simulink model "Wind_App"  (R2020a)
settings: Solver=VariableStepAuto  StartTime=0.0  StopTime=10  RelTol=1e-3
undefined symbols (not defined in the file): D1, D11, Delta
libraries: powerlib x15, re_lib x1
settings Model: Creator=royde  LastModifiedBy=royde

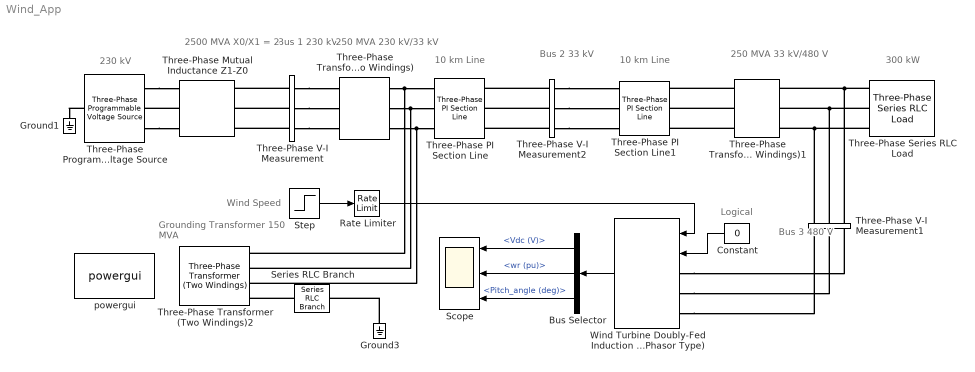
== system Wind_App ==
  note: Bus 1
      | 230 kV
  note: 230 kV
  note: 2500 MVA
      | X0/X1 = 2
  note: 250 MVA
      | 230 kV/33 kV
  note: 250 MVA
      | 33 kV/480 V
  note: Bus 3
      | 480 V
  note: 300 kW
  note: Wind Speed
  note: Logical
  note: Bus 2
      | 33 kV
  note: 10 km Line
  note: 10 km Line
  note: Grounding Transformer
      | 150 MVA
  Bus Selector : BusSelector  OutputSignals=Vdc (V),wr (pu),Pitch_angle (deg)
  Constant : Constant  Value=0
  Ground1 : powerlib/Elements/Ground  LConnTagsString=a
  Ground3 : powerlib/Elements/Ground  LConnTagsString=a
      settings: SourceProductBaseCode=MT,PS
  Rate Limiter : RateLimiter
  Scope : Scope  NumInputPorts=3
  Series RLC Branch : powerlib/Elements/Series RLC Branch  LConnTagsString=__new0  RConnTagsString=__new0  BranchType=R  Resistance=3.5  Inductance=1e-3  SetiL0=off  InitialCurrent=0  Capacitance=1e-6  Setx0=off  InitialVoltage=0  Measurements=None
  Step : Step  Time=5  Before=8  After=14  SampleTime=0
  Three-Phase Mutual Inductance Z1-Z0 : powerlib/Elements/Three-Phase Mutual Inductance Z1-Z0  LConnTagsString=a|b|c  RConnTagsString=A|B|C  PositiveSequence="[0.2  1/(2*pi*60)]*230e3^2/2500e6"  ZeroSequence="[0.4  2/(2*pi*60)]*230e3^2/2500e6"
      settings: SourceProductBaseCode=PS
  Three-Phase PI Section Line : powerlib/Elements/Three-Phase PI Section Line  LConnTagsString=a|b|c  RConnTagsString=A|B|C  Frequency=60  Resistances=[ 0.01273 0.3864]  Inductances="[ 0.9337e-3  4.1264e-3]"  Capacitances=[12.74e-9 7.751e-9]  Length=10
  Three-Phase PI Section Line1 : powerlib/Elements/Three-Phase PI Section Line  LConnTagsString=a|b|c  RConnTagsString=A|B|C  Frequency=60  Resistances=[ 0.01273 0.3864]  Inductances="[ 0.9337e-3  4.1264e-3]"  Capacitances=[12.74e-9 7.751e-9]  Length=10
  Three-Phase Programmable Voltage Source : powerlib/Electrical Sources/Three-Phase Programmable Voltage Source  PositiveSequence="[230e3  0 60]"  VariationEntity=None  VariationType=Table of time-amplitude pairs  VariationTypeAlt=Step  VariationStep=0.5  VariationRate=10  VariationMagnitude=0.3  VariationFrequency=2  VariationTiming=[1 2]  VariationPhaseA=off  Amplitudes=[1 0.8 1.2 1.0]  TimeValues=[0 0.1 0.15 0.2]  HarmonicGeneration=off  HarmonicA=[3 0.2 -25 0]  HarmonicB=[2 0.15 35 2]  Timing="[0.05  3]"  BusType=swing  Pref=0  Qref=0  Qmin=-inf  Qmax=inf
  Three-Phase Series RLC Load : powerlib/Elements/Three-Phase Series RLC Load  LConnTagsString=A|B|C  Configuration=Y (grounded)  NominalVoltage=480  Vabc=[1e3 1e3 1e3]  Vabcp=[1e3 1e3 1e3]  NominalFrequency=60  UnbalancedPower=off  ActivePower=300e3  InductivePower=0  CapacitivePower=0  Pabc=[10e3 9e3 11e3]  QLabc=[100 90 110]  QCabc=[100 90 110]  Pabcp=[10e3 9e3 11e3]  QLabcp=[100 90 110]  QCabcp=[100 90 110]  Measurements=None  LoadType=constant Z
  Three-Phase Transformer (Two Windings) : powerlib/Elements/Three-Phase Transformer (Two Windings)  Winding1Connection=Yg  Winding2Connection=Delta (D1)  CoreType=Three single-phase transformers  SetSaturation=off  Hysteresis=off  DataFile='hysteresis'  SetInitialFlux=off  Measurements=None  UNITS=pu  NominalPower=[ 250e6 , 60 ]  Winding1=[ 230e3 , 0.002 , 0.08 ]  Winding2=[ 33e3 , 0.002 , 0.08 ]  Rm=500  Lm=500  L0=0.5  Saturation=[ 0,0 ; 0.0024,1.2 ; 1.0,1.52 ]  InitialFluxes=[ 0.8 , -0.8 , 0.7 ]  BreakLoop=off  DiscreteSolver=Trapezoidal iterative  DataType=off  TransfoNumber=1
  Three-Phase Transformer (Two Windings)1 : powerlib/Elements/Three-Phase Transformer (Two Windings)  Winding1Connection=Yg  Winding2Connection=Delta (D1)  CoreType=Three single-phase transformers  SetSaturation=off  Hysteresis=off  DataFile='hysteresis'  SetInitialFlux=off  Measurements=None  UNITS=pu  NominalPower=[ 250e6 , 60 ]  Winding1=[ 33e3 , 0.002 , 0.08 ]  Winding2=[ 480e3 , 0.002 , 0.08 ]  Rm=500  Lm=inf  L0=0.5  Saturation=[ 0,0 ; 0.0024,1.2 ; 1.0,1.52 ]  InitialFluxes=[ 0.8 , -0.8 , 0.7 ]  BreakLoop=off  DiscreteSolver=Trapezoidal iterative  DataType=off  TransfoNumber=1
  Three-Phase Transformer (Two Windings)2 : powerlib/Elements/Three-Phase Transformer (Two Windings)  Winding1Connection=Yn  Winding2Connection=Delta (D11)  CoreType=Three single-phase transformers  SetSaturation=off  Hysteresis=off  DataFile='hysteresis'  SetInitialFlux=off  Measurements=None  UNITS=pu  NominalPower=[ 150e6 , 60 ]  Winding1=[ 33e3 , 4.5/(33e3^2/150e6)/30 , 4.5/(33e3^2/150e6) ]  Winding2=[ 33e3 , 0.000002 , 0 ]  Rm=500  Lm=500  L0=0.5  Saturation=[ 0,0 ; 0.0024,1.2 ; 1.0,1.52 ]  InitialFluxes=[ 0.8 , -0.8 , 0.7 ]  BreakLoop=off  DiscreteSolver=Trapezoidal iterative  DataType=off  TransfoNumber=1
  Three-Phase V-I Measurement : powerlib/Measurements/Three-Phase V-I Measurement  VoltageMeasurement=phase-to-ground  SetLabelV=on  LabelV=Vabc_Bus1  Vpu=on  VpuLL=off  CurrentMeasurement=no  SetLabelI=off  LabelI=Iabc  Ipu=off  Pbase=100e6  Vbase=230e3  OutputType=Complex  PhasorSimulation=on  PSBequivalent=0
  Three-Phase V-I Measurement1 : powerlib/Measurements/Three-Phase V-I Measurement  VoltageMeasurement=phase-to-ground  SetLabelV=on  LabelV=Vabc_Bus3  Vpu=on  VpuLL=off  CurrentMeasurement=yes  SetLabelI=on  LabelI=Iabc_Bus2  Ipu=on  Pbase=100e6  Vbase=480  OutputType=Complex  PhasorSimulation=on  PSBequivalent=0
  Three-Phase V-I Measurement2 : powerlib/Measurements/Three-Phase V-I Measurement  VoltageMeasurement=phase-to-ground  SetLabelV=on  LabelV=Vabc_Bus2  Vpu=on  VpuLL=off  CurrentMeasurement=no  SetLabelI=off  LabelI=Iabc  Ipu=off  Pbase=100e6  Vbase=33e3  OutputType=Complex  PhasorSimulation=on  PSBequivalent=0
  Wind Turbine Doubly-Fed Induction Generator (Phasor Type) : re_lib/Wind Generation/Wind Turbine Doubly-Fed Induction Generator (Phasor Type)  ExternalTm=off  nom=[6*1.5e6/0.9 575 60]  sta=[ 0.00706 0.171]  rot=[ 0.005 0.156]  Lm=2.9  mec=[5.04 0.01 3]  init=[0.2 0 0 0 0 0]  speed_power=[0 0; 0.24 0.007; 0.36 0.024; 0.6 0.112; 0.96 0.46; 1.2 0.898; 1.5 0.898]  Pmec=6*1.5e6  speed_ABCD=[0.7 0.71 1.2 1.21]  power_C=0.73  wind_point_C=12  pitch_gain=500  pitch_max=45  pitch_rate=2  Pmax=0.5  Lchoke=[0.15 0.15/100]  init_inductor=[0 90]  Vdc_nom=1200  capacitor=6*10000e-6  ControlVQ=Voltage regulation  Vref=1.0  ExternalVref=off  Qref=0  ExternalQref=off  Iq_ref=0  ExternalIqref=off  Kpi_volt_reg=[1.25 300]  Xs=0.02  Kpi_Q=[0.05 5]  Kpi_power_reg=[1 100]  Kpi_dc_reg=[0.002 0.05]  Kpi_grid_side_cur_reg=[1 100]  Kpi_rotor_side_cur_reg=[0.3 8]  V_slew_rate=100  Q_slew_rate=100  power_slew_rate=1  current_slew_rate=200
      settings: SourceProductBaseCode=PS
  powergui : powerlib/powergui  Priority=2  SimulationMode=Phasor  SampleTime=0  frequency=60  Iterations=50  frequencyindice=60  Pbase=100e6  ErrMax=1e-4  UnitsV=kV  UnitsW=MW  buscounter=0  FunctionMessages=off  echomessages=off  EnableUseOfTLC=off  CurrentSourceSwitches=off  DisableSnubberDevices=off  DisableRonSwitches=off  DisableVfSwitches=off  DisplayEquations=off  AutomaticDiscreteSolvers=off  SolverType=Tustin  Interpol=off  ExternalGateDelay=off  methode=off  Ts=0  x0status=blocks  SPID=off  SwTol=0  HookPort=off  NonlinearTolerance=1e-4  nMaxIteration=100  ContinueOnMaxIteration=off  RestoreLinks=warning  ResistiveCurrentMeasurement=off  Frange=[0:2:500]  Ylog=off  Xlog=off  ShowGrid=off  save=off  variable=ZData  structure=0  ZoomFFT=on  StartTime=0.0  cycles=1  DisplayStyle=1  fundamental=60  FreqAxis=off  MaxFrequency=1000  frequencyindicesteady=1  RmsSteady=1  display=off
  wires:
  Step/1 -> Rate Limiter/1
  Wind Turbine Doubly-Fed Induction Generator (Phasor Type)/1 -> Bus Selector/1
  Rate Limiter/1 -> Wind Turbine Doubly-Fed Induction Generator (Phasor Type)/1
  Constant/1 -> Wind Turbine Doubly-Fed Induction Generator (Phasor Type)/2
  Bus Selector/1 -> Scope/1  "<Vdc (V)>"
  Bus Selector/2 -> Scope/2  "<wr (pu)>"
  Bus Selector/3 -> Scope/3  "<Pitch_angle (deg)>"
  connections:
  Three-Phase Programmable Voltage Source/LConn1 -- Ground1/LConn1
  Three-Phase Mutual Inductance Z1-Z0/LConn2 -- Three-Phase Programmable Voltage Source/RConn2
  Three-Phase Programmable Voltage Source/RConn1 -- Three-Phase Mutual Inductance Z1-Z0/LConn1
  Three-Phase Programmable Voltage Source/RConn3 -- Three-Phase Mutual Inductance Z1-Z0/LConn3
  Three-Phase V-I Measurement/LConn1 -- Three-Phase Mutual Inductance Z1-Z0/RConn1
  Three-Phase V-I Measurement/LConn2 -- Three-Phase Mutual Inductance Z1-Z0/RConn2
  Three-Phase V-I Measurement/LConn3 -- Three-Phase Mutual Inductance Z1-Z0/RConn3
  Three-Phase V-I Measurement/RConn1 -- Three-Phase Transformer (Two Windings)/LConn1
  Three-Phase V-I Measurement/RConn2 -- Three-Phase Transformer (Two Windings)/LConn2
  Three-Phase V-I Measurement/RConn3 -- Three-Phase Transformer (Two Windings)/LConn3
  Three-Phase V-I Measurement1/LConn1 -- Three-Phase Series RLC Load/LConn1 -- Three-Phase Transformer (Two Windings)1/RConn1
  Three-Phase V-I Measurement1/LConn2 -- Three-Phase Series RLC Load/LConn2 -- Three-Phase Transformer (Two Windings)1/RConn2
  Three-Phase V-I Measurement1/LConn3 -- Three-Phase Series RLC Load/LConn3 -- Three-Phase Transformer (Two Windings)1/RConn3
  Three-Phase Transformer (Two Windings)/RConn1 -- Three-Phase Transformer (Two Windings)2/LConn1 -- Three-Phase PI Section Line/LConn1
  Three-Phase Transformer (Two Windings)/RConn2 -- Three-Phase Transformer (Two Windings)2/LConn2 -- Three-Phase PI Section Line/LConn2
  Three-Phase Transformer (Two Windings)/RConn3 -- Three-Phase Transformer (Two Windings)2/LConn3 -- Three-Phase PI Section Line/LConn3
  Three-Phase V-I Measurement2/LConn1 -- Three-Phase PI Section Line/RConn1
  Three-Phase V-I Measurement2/LConn2 -- Three-Phase PI Section Line/RConn2
  Three-Phase V-I Measurement2/LConn3 -- Three-Phase PI Section Line/RConn3
  Three-Phase V-I Measurement2/RConn1 -- Three-Phase PI Section Line1/LConn1
  Three-Phase V-I Measurement2/RConn2 -- Three-Phase PI Section Line1/LConn2
  Three-Phase V-I Measurement2/RConn3 -- Three-Phase PI Section Line1/LConn3
  Three-Phase Transformer (Two Windings)1/LConn1 -- Three-Phase PI Section Line1/RConn1
  Three-Phase Transformer (Two Windings)1/LConn2 -- Three-Phase PI Section Line1/RConn2
  Three-Phase Transformer (Two Windings)1/LConn3 -- Three-Phase PI Section Line1/RConn3
  Wind Turbine Doubly-Fed Induction Generator (Phasor Type)/LConn1 -- Three-Phase V-I Measurement1/RConn1
  Wind Turbine Doubly-Fed Induction Generator (Phasor Type)/LConn2 -- Three-Phase V-I Measurement1/RConn2
  Wind Turbine Doubly-Fed Induction Generator (Phasor Type)/LConn3 -- Three-Phase V-I Measurement1/RConn3
  Series RLC Branch/LConn1 -- Three-Phase Transformer (Two Windings)2/LConn4
  Ground3/LConn1 -- Series RLC Branch/RConn1
